simulink model "pmsmscratchmodel"  (R2021a)
settings: Solver=VariableStepAuto  StartTime=0.0  StopTime=5  RelTol=1e-3
libraries: simulink x12
settings Model: MinMaxOverflowLogging=ForceOff  Creator=Prince  LastModifiedBy=rahul
settings SolverCC: AlgebraicLoopSolver=TrustRegion
settings DebuggingCC: SFMachineParentedDataDiag=warning

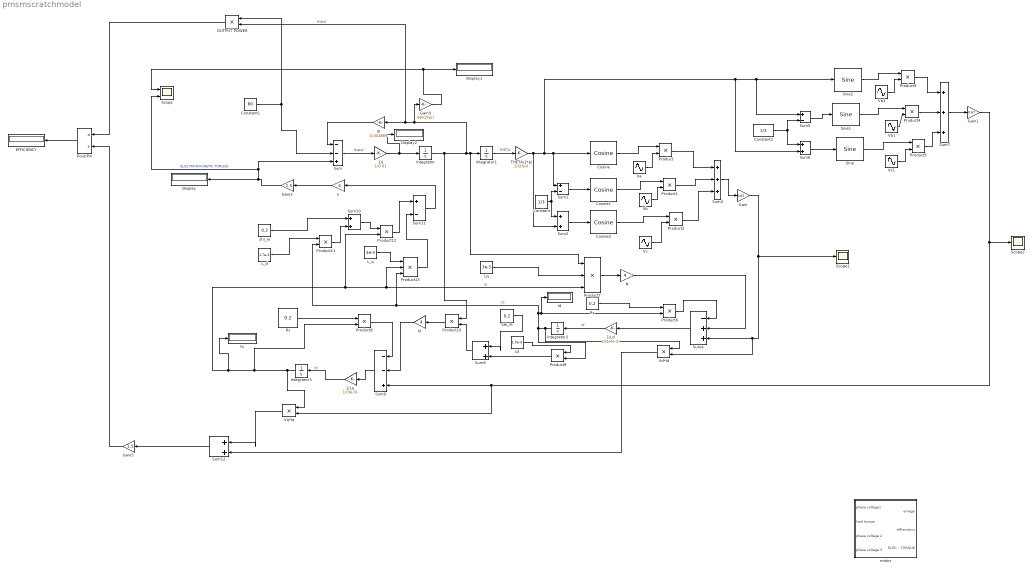
== system pmsmscratchmodel ==
  1/J : Gain  Gain=1/0.01
  "1/Ld " : Gain  Gain=1/(1.7e-3)
  "1/Lq " : Gain  Gain=1/(3e-3)
  B : Gain  Gain=0.001889
  Constant : Constant  Value=1/3
  Constant1 : Constant  Value=80
  Constant2 : Constant  Value=1/3
  Cosine : simulink/Lookup Tables/Cosine  Formula=cos(2*pi*u)  NumDataPoints=(2^5)+1  OutputWordLength=16  InternalRulePriority=Speed
      settings: SourceProductBaseCode=SL
  Cosine1 : simulink/Lookup Tables/Cosine  Formula=cos(2*pi*u)  NumDataPoints=(2^5)+1  OutputWordLength=16  InternalRulePriority=Speed
      settings: SourceProductBaseCode=SL
  Cosine2 : simulink/Lookup Tables/Cosine  Formula=cos(2*pi*u)  NumDataPoints=(2^5)+1  OutputWordLength=16  InternalRulePriority=Speed
      settings: SourceProductBaseCode=SL
  Display : Display
  Display1 : Display
  Display2 : Display
  EFFICIENCY : Display
  Gain : Gain  Gain=0.67
  Gain1 : Gain  Gain=-0.67
  Gain2 : Gain  Gain=1.5
  Gain3 : Gain  Gain=60/(2*pi)
  Gain5 : Gain  Gain=1.5
  Id : Display
  Integrator{,1..3} (4 alike) : Integrator
  "Iq " : Display
  L_d : Constant  Value=1.7e-3
  "L_q " : Constant  Value=3e-3
  Ld : Constant  Value=1.7e-3
  Lq : Constant  Value=3e-3
  N : Gain  Gain=4
  "N " : Gain  Gain=4
  OUTPUT POWER : Product
  Pout/Pin : Product  Inputs=*/
  Product{,1..6,8..12} (12 alike) : Product
  Product13 : Product  Inputs=3
  Product7 : Product  Inputs=3
  Rs : Constant  Value=0.2
  "Rs " : Constant  Value=0.2
  SHI_M : Constant  Value=0.2
  Scope : Scope  NumInputPorts=2
  Scope1 : Scope
  Scope2 : Scope
  Sine : simulink/Lookup Tables/Sine  Formula=sin(2*pi*u)  NumDataPoints=(2^5)+1  OutputWordLength=16  InternalRulePriority=Speed
  Sine1 : simulink/Lookup Tables/Sine  Formula=sin(2*pi*u)  NumDataPoints=(2^5)+1  OutputWordLength=16  InternalRulePriority=Speed
  Sine2 : simulink/Lookup Tables/Sine  Formula=sin(2*pi*u)  NumDataPoints=(2^5)+1  OutputWordLength=16  InternalRulePriority=Speed
  Sum : Sum  Inputs=--+
  Sum1 : Sum  Inputs=+-
  Sum10 : Sum  Inputs=|++
  Sum11 : Sum  Inputs=+-
  Sum12 : Sum  Inputs=|++
  Sum2 : Sum
  Sum3 : Sum  Inputs=+++
  Sum4 : Sum  Inputs=-++
  Sum5 : Sum  Inputs=+-
  Sum6 : Sum
  Sum7 : Sum  Inputs=+++
  Sum8 : Sum  Inputs=|++
  Sum9 : Sum  Inputs=--+
  THETA/2*pi : Gain  Gain=1/(2*pi)
  Va : Sin  Amplitude=200  Frequency=2*pi*50  SampleTime=0
  Va1 : Sin  Amplitude=200  Frequency=2*pi*50  SampleTime=0
  Vb : Sin  Amplitude=200  Frequency=2*pi*50  Phase=((-2)*pi)/3  SampleTime=0
  Vb1 : Sin  Amplitude=200  Frequency=2*pi*50  Phase=((-2)*pi)/3  SampleTime=0
  Vc : Sin  Amplitude=200  Frequency=2*pi*50  Phase=(2*pi)/3  SampleTime=0
  "Vc1 " : Sin  Amplitude=200  Frequency=2*pi*50  Phase=(2*pi)/3  SampleTime=0
  Vd*Id : Product
  Vq*Iq : Product
  motor : Subsystem
  n : Gain  Gain=4
  shi_m : Constant  Value=0.2
  wires:
  Integrator/1 -> Product10/1, Product7/1, Integrator1/1, Gain3/1, OUTPUT POWER/2, B/1  "theta'"
  Sum/1 -> 1/J/1  "theta''"
  Constant1/1 -> Sum/2, OUTPUT POWER/1
  B/1 -> Sum/1
  1/J/1 -> Display2/1, Integrator/1
  THETA/2*pi/1 -> Sum2/2, Sum6/2, Sum5/1, Sine2/1, Sum1/1, Cosine/1
  Integrator1/1 -> THETA/2*pi/1  "THETA"
  Sum1/1 -> Cosine1/1
  Sum2/1 -> Cosine2/1
  Cosine/1 -> Product/1
  Va/1 -> Product/2
  Cosine1/1 -> Product1/1
  Cosine2/1 -> Product2/1
  Product/1 -> Sum3/1
  Product1/1 -> Sum3/2
  Product2/1 -> Sum3/3
  Sum3/1 -> Gain/1
  Va1/1 -> Product3/2
  Sum5/1 -> Sine1/1
  Sine1/1 -> Product4/1
  Sum6/1 -> Sine/1
  Sine/1 -> Product5/1
  Sine2/1 -> Product3/1
  Product3/1 -> Sum7/1
  Product4/1 -> Sum7/2
  Product5/1 -> Sum7/3
  Sum7/1 -> Gain1/1
  "1/Ld "/1 -> Integrator2/1  "Id'"
  "1/Lq "/1 -> Integrator3/1  "Iq'"
  "Rs "/1 -> Product6/1
  Integrator2/1 -> Vd*Id/1, Product11/2, Product13/3, Product6/2, Id/1, Product9/2  "Id"
  Integrator3/1 -> Vq*Iq/1, "Iq "/1, Product7/3, Product13/2, Product12/2, Product8/2  "Iq"
  Lq/1 -> Product7/2
  Product7/1 -> "N "/1
  Gain/1 -> Sum4/3, Vd*Id/2, Scope1/1
  "N "/1 -> Sum4/2
  Product6/1 -> Sum4/1
  Sum4/1 -> "1/Ld "/1
  Rs/1 -> Product8/1
  Ld/1 -> Product9/1
  Product9/1 -> Sum8/2
  SHI_M/1 -> Sum8/1
  Sum8/1 -> Product10/2
  Product10/1 -> N/1
  Gain1/1 -> Vq*Iq/2, Sum9/3, Scope2/1
  N/1 -> Sum9/2
  Product8/1 -> Sum9/1
  Sum9/1 -> "1/Lq "/1
  L_d/1 -> Product11/1
  shi_m/1 -> Sum10/1
  Product11/1 -> Sum10/2
  Sum10/1 -> Product12/1
  "L_q "/1 -> Product13/1
  Product13/1 -> Sum11/2
  Product12/1 -> Sum11/1
  Sum11/1 -> n/1
  n/1 -> Gain2/1
  Gain2/1 -> Scope/2, Sum/3, Display/1  "ELECTROMAGNETIC TORQUE"
  Gain3/1 -> Scope/1, Display1/1
  Vd*Id/1 -> Sum12/2
  Vq*Iq/1 -> Sum12/1
  Sum12/1 -> Gain5/1
  OUTPUT POWER/1 -> Pout/Pin/1
  Gain5/1 -> Pout/Pin/2
  Pout/Pin/1 -> EFFICIENCY/1
  Vb/1 -> Product1/2
  Vc/1 -> Product2/2
  Vb1/1 -> Product4/2
  "Vc1 "/1 -> Product5/2
  Constant/1 -> Sum1/2, Sum2/1
  Constant2/1 -> Sum6/1, Sum5/2

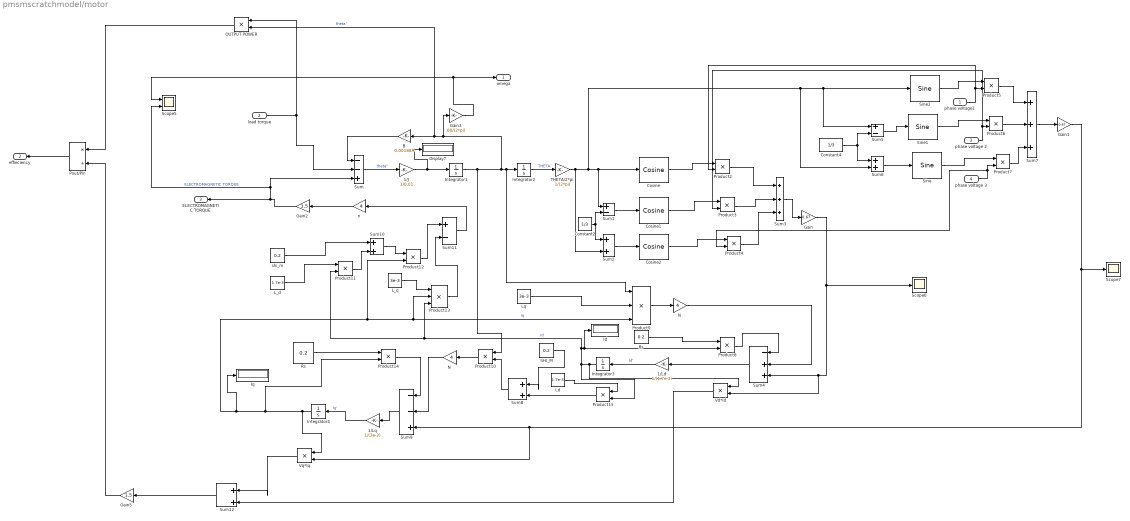
== system pmsmscratchmodel/motor ==
  "phase voltage1 " : Inport
  load torque : Inport  Port=2
  phase voltage 2 : Inport  Port=3
  phase voltage 3 : Inport  Port=4
  1/J : Gain  Gain=1/0.01
  "1/Ld " : Gain  Gain=1/(1.7e-3)
  "1/Lq " : Gain  Gain=1/(3e-3)
  B : Gain  Gain=0.001889
  Constant2 : Constant  Value=1/3
  Constant4 : Constant  Value=1/3
  Cosine : simulink/Lookup Tables/Cosine  Formula=cos(2*pi*u)  NumDataPoints=(2^5)+1  OutputWordLength=16  InternalRulePriority=Speed
      settings: SourceProductBaseCode=SL
  Cosine1 : simulink/Lookup Tables/Cosine  Formula=cos(2*pi*u)  NumDataPoints=(2^5)+1  OutputWordLength=16  InternalRulePriority=Speed
      settings: SourceProductBaseCode=SL
  Cosine2 : simulink/Lookup Tables/Cosine  Formula=cos(2*pi*u)  NumDataPoints=(2^5)+1  OutputWordLength=16  InternalRulePriority=Speed
      settings: SourceProductBaseCode=SL
  Display7 : Display
  Gain : Gain  Gain=0.67
  Gain1 : Gain  Gain=-0.67
  Gain2 : Gain  Gain=1.5
  Gain3 : Gain  Gain=60/(2*pi)
  Gain5 : Gain  Gain=1.5
  Id : Display
  Integrator{1..4} (4 alike) : Integrator
  "Iq " : Display
  L_d : Constant  Value=1.7e-3
  "L_q " : Constant  Value=3e-3
  Ld : Constant  Value=1.7e-3
  Lq : Constant  Value=3e-3
  N : Gain  Gain=4
  "N " : Gain  Gain=4
  OUTPUT POWER : Product
  Pout/Pin : Product  Inputs=*/
  Product{2..8,10..12,14..15} (12 alike) : Product
  Product13 : Product  Inputs=3
  Product9 : Product  Inputs=3
  Rs : Constant  Value=0.2
  "Rs " : Constant  Value=0.2
  SHI_M : Constant  Value=0.2
  Scope5 : Scope  NumInputPorts=2
  Scope6 : Scope
  Scope7 : Scope
  Sine : simulink/Lookup Tables/Sine  Formula=sin(2*pi*u)  NumDataPoints=(2^5)+1  OutputWordLength=16  InternalRulePriority=Speed
  Sine1 : simulink/Lookup Tables/Sine  Formula=sin(2*pi*u)  NumDataPoints=(2^5)+1  OutputWordLength=16  InternalRulePriority=Speed
  Sine2 : simulink/Lookup Tables/Sine  Formula=sin(2*pi*u)  NumDataPoints=(2^5)+1  OutputWordLength=16  InternalRulePriority=Speed
  Sum : Sum  Inputs=--+
  Sum1 : Sum  Inputs=+-
  Sum10 : Sum  Inputs=|++
  Sum11 : Sum  Inputs=+-
  Sum12 : Sum  Inputs=|++
  Sum2 : Sum
  Sum3 : Sum  Inputs=+++
  Sum4 : Sum  Inputs=-++
  Sum5 : Sum  Inputs=+-
  Sum6 : Sum
  Sum7 : Sum  Inputs=+++
  Sum8 : Sum  Inputs=|++
  Sum9 : Sum  Inputs=--+
  THETA/2*pi : Gain  Gain=1/(2*pi)
  Vd*Id : Product
  Vq*Iq : Product
  n : Gain  Gain=4
  shi_m : Constant  Value=0.2
  omega : Outport
  effieciency : Outport  Port=2
  ELECTROMAGNETIC TORQUE : Outport  Port=3
  wires:
  Constant2/1 -> Sum1/2, Sum2/1
  Sum/1 -> 1/J/1  "theta''"
  Gain2/1 -> ELECTROMAGNETIC TORQUE/1, Scope5/2, Sum/3  "ELECTROMAGNETIC TORQUE"
  Product2/1 -> Sum3/1
  Sum3/1 -> Gain/1
  SHI_M/1 -> Sum8/1
  Integrator1/1 -> Product10/1, Product9/1, Integrator2/1, Gain3/1, OUTPUT POWER/2, B/1  "theta'"
  Product14/1 -> Sum9/1
  Constant4/1 -> Sum6/1, Sum5/2
  Sum2/1 -> Cosine2/1
  L_d/1 -> Product11/1
  Gain3/1 -> omega/1, Scope5/1
  Product3/1 -> Sum3/2
  shi_m/1 -> Sum10/1
  Product13/1 -> Sum11/2
  Integrator2/1 -> THETA/2*pi/1  "THETA"
  Sum11/1 -> n/1
  Rs/1 -> Product14/1
  Vq*Iq/1 -> Sum12/1
  Sum7/1 -> Gain1/1
  OUTPUT POWER/1 -> Pout/Pin/1
  Sum9/1 -> "1/Lq "/1
  "L_q "/1 -> Product13/1
  Sum1/1 -> Cosine1/1
  Sum6/1 -> Sine/1
  Sum10/1 -> Product12/1
  Product7/1 -> Sum7/3
  Sum8/1 -> Product10/2
  1/J/1 -> Display7/1, Integrator1/1
  Gain/1 -> Sum4/3, Vd*Id/2, Scope6/1
  THETA/2*pi/1 -> Sum2/2, Sum6/2, Sum5/1, Sine2/1, Sum1/1, Cosine/1
  Sum5/1 -> Sine1/1
  Ld/1 -> Product15/1
  "phase voltage1 "/1 -> Product2/2, Product5/2
  Sine2/1 -> Product5/1
  Product11/1 -> Sum10/2
  Sum12/1 -> Gain5/1
  Gain5/1 -> Pout/Pin/2
  "Rs "/1 -> Product8/1
  Integrator3/1 -> Vd*Id/1, Product11/2, Product13/3, Product8/2, Id/1, Product15/2  "Id"
  Integrator4/1 -> Vq*Iq/1, "Iq "/1, Product9/3, Product13/2, Product12/2, Product14/2  "Iq"
  Cosine2/1 -> Product4/1
  Sine1/1 -> Product6/1
  Gain1/1 -> Vq*Iq/2, Sum9/3, Scope7/1
  Product8/1 -> Sum4/1
  B/1 -> Sum/1
  "N "/1 -> Sum4/2
  n/1 -> Gain2/1
  Product10/1 -> N/1
  load torque/1 -> Sum/2, OUTPUT POWER/1
  Sine/1 -> Product7/1
  Cosine/1 -> Product2/1
  Lq/1 -> Product9/2
  N/1 -> Sum9/2
  "1/Ld "/1 -> Integrator3/1  "Id'"
  Product6/1 -> Sum7/2
  Sum4/1 -> "1/Ld "/1
  "1/Lq "/1 -> Integrator4/1  "Iq'"
  Product15/1 -> Sum8/2
  Vd*Id/1 -> Sum12/2
  Product12/1 -> Sum11/1
  Product4/1 -> Sum3/3
  Product5/1 -> Sum7/1
  Cosine1/1 -> Product3/1
  Product9/1 -> "N "/1
  phase voltage 2/1 -> Product3/2, Product6/2
  Pout/Pin/1 -> effieciency/1
  phase voltage 3/1 -> Product4/2, Product7/2
